simulink model "car_model"  (R2017a)
settings: Solver=ode8  StartTime=0.0  StopTime=tf  FixedStep=1e-3  RelTol=1e-3  AbsTol=1e-6
values from neighbouring files (symbols this model uses):
  sys = kinematic_model(sys)    [load_kin.m]
undefined symbols (not defined in the file or in its folder): L, MAX_DELTA, w, x0
(part 2 of 2)

== matlab function car_model/Vehicle/Steering_model/Efforts/Constrained_efforts ==
  data: in1 input; in2 input; fs output
function fs = ConstrainedEffort(in1,in2)

%    This function was generated by the Symbolic Math Toolbox version 7.2.

%    11-Nov-2020 11:00:39



delta_o = in1(5,:);

f_phi_i = in2(1,:);

f_phi_l = in2(4,:);

f_phi_o = in2(2,:);

f_phi_r = in2(3,:);

p1 = in1(10,:);

p2 = in1(11,:);

p3 = in1(12,:);

p4 = in1(13,:);

phi_i = in1(6,:);

phi_l = in1(9,:);

phi_o = in1(7,:);

phi_r = in1(8,:);

theta = in1(3,:);

t2 = p1.^2;

t3 = tan(theta);

t4 = p4.^2;

t5 = theta.*2.0;

t6 = p3.^2;

t7 = delta_o.*2.0;

t8 = phi_o.*2.0;

t9 = p2.^2;

t10 = t5+t7+t8;

t11 = sin(t10);

t12 = t5+t7-t8;

t13 = sin(t12);

t14 = phi_o.*4.0;

t15 = t5+t7+t14;

t16 = sin(t15);

t17 = sin(t5);

t18 = t5+t7;

t19 = sin(t18);

t20 = phi_l.*2.0;

t21 = phi_l.*4.0;

t22 = -t5+t20;

t23 = sin(t22);

t24 = t5+t20;

t25 = sin(t24);

t26 = phi_l.*3.0;

t27 = phi_r.*2.0;

t28 = phi_r.*4.0;

t29 = delta_o-t14+theta;

t30 = sin(t29);

t31 = delta_o+t14+theta;

t32 = sin(t31);

t33 = phi_o.*3.0;

t34 = t3.*(3.0./2.0);

t35 = t34+9.0./2.0;

t36 = 1.0./t35;

t37 = t3.*t36.*(9.0./2.0);

t38 = atan(t37);

t39 = t38.*2.0;

t40 = delta_o+theta;

t41 = sin(t40);

t42 = phi_i.*4.0;

t43 = t3.*t36.*(2.7e1./4.0);

t44 = t43+9.0./2.0;

t45 = 1.0./t44.^2;

t46 = t21+theta;

t47 = sin(t46);

t48 = t5+t7-t14;

t49 = sin(t48);

t50 = sin(t8);

t51 = sin(t14);

t52 = -t5+t27;

t53 = sin(t52);

t54 = t5+t27;

t55 = sin(t54);

t56 = phi_r.*3.0;

t57 = t21-theta;

t58 = sin(t57);

t59 = -t5+t21;

t60 = sin(t59);

t61 = t5+t21;

t62 = sin(t61);

t63 = cos(theta);

t64 = sin(theta);

t65 = phi_i.*2.0;

t69 = cos(t39);

t70 = t69.*(9.0./2.0);

t71 = sin(t39);

t72 = t71.*(3.0./2.0);

t66 = t70+t72+9.0./2.0;

t67 = t5+t39+t65;

t68 = sin(t67);

t73 = t66.^2;

t74 = cos(t7);

t75 = t74.*(9.0./2.0);

t76 = sin(t7);

t79 = t76.*(3.0./2.0);

t77 = t75-t79+9.0./2.0;

t78 = 1.0./t77.^2;

t80 = t5+t39+t42;

t81 = sin(t80);

t82 = t5+t39;

t83 = sin(t82);

t84 = t38-t42+theta;

t85 = sin(t84);

t86 = t38+t42+theta;

t87 = sin(t86);

t88 = t28+theta;

t89 = sin(t88);

t90 = t38+theta;

t91 = sin(t90);

t92 = 1.0./t44;

t93 = t28-theta;

t94 = sin(t93);

t95 = -t5+t28;

t96 = sin(t95);

t97 = t5+t28;

t98 = sin(t97);

t99 = t5+t39-t65;

t100 = sin(t99);

t101 = 1.0./t77;

t102 = t5+t39-t42;

t103 = sin(t102);

t104 = t3.^2;

t105 = 1.0./t35.^2;

t106 = t104.*t105.*(8.1e1./4.0);

t107 = t106+1.0;

t108 = 1.0./sqrt(t107);

t110 = t108.*9.0;

t111 = t3.*t36.*t108.*(2.7e1./4.0);

t109 = t110-t111;

t112 = cos(delta_o);

t113 = 1.0./t112.^2;

t114 = 1.0./t107;

t115 = t109.^2;

t116 = t110+t111;

t117 = 1.0./t116.^2;

t118 = phi_i.*3.0;

t119 = 1.0./t112;

t120 = 1.0./t116;

t121 = sin(t65);

t122 = sin(t42);

t123 = phi_o+t5+t7;

t124 = sin(t123);

t125 = t6.*t124.*3.888459953911314e-2;

t126 = delta_o+phi_o+theta;

t127 = sin(t126);

t128 = -phi_o+t5+t7;

t129 = sin(t128);

t130 = t6.*t129.*3.888459953911314e-2;

t131 = t2.*t16.*6.480766589852189e-3;

t132 = t9.*t49.*6.480766589852189e-3;

t133 = t9.*t16.*6.480766589852189e-3;

t134 = t5+t7+t33;

t135 = sin(t134);

t136 = t2.*t19.*3.888459953911314e-2;

t137 = t9.*t19.*3.888459953911314e-2;

t138 = t6.*t19.*5.184613271881752e-2;

t139 = delta_o-phi_o+theta;

t140 = sin(t139);

t141 = t2.*t30.*1.296153317970438e-2;

t142 = t2.*t32.*1.296153317970438e-2;

t143 = t9.*t30.*1.296153317970438e-2;

t144 = t9.*t32.*1.296153317970438e-2;

t145 = delta_o-t33+theta;

t146 = sin(t145);

t147 = delta_o+t33+theta;

t148 = sin(t147);

t149 = t2.*t81.*6.480766589852189e-3;

t150 = t2.*t83.*3.888459953911314e-2;

t151 = t2.*t85.*1.296153317970438e-2;

t152 = t2.*t87.*1.296153317970438e-2;

t153 = t9.*t73.*t78.*t103.*6.480766589852189e-3;

t154 = t9.*t73.*t78.*t81.*6.480766589852189e-3;

t155 = t9.*t73.*t78.*t83.*3.888459953911314e-2;

t156 = t9.*t73.*t78.*t85.*1.296153317970438e-2;

t157 = t9.*t73.*t78.*t87.*1.296153317970438e-2;

t158 = p1.*p2.*t66.*t101.*t103.*1.296153317970438e-2;

t159 = p1.*p2.*t66.*t81.*t101.*1.296153317970438e-2;

t160 = p1.*p2.*t66.*t83.*t101.*7.776919907822627e-2;

t161 = p1.*p2.*t66.*t85.*t101.*2.592306635940876e-2;

t162 = p1.*p2.*t66.*t87.*t101.*2.592306635940876e-2;

t163 = t6.*t83.*t113.*t114.*t115.*t117.*5.184613271881752e-2;

t164 = -phi_i+t38+theta;

t165 = sin(t164);

t166 = t38+t118+theta;

t167 = sin(t166);

t168 = phi_i+t5+t39;

t169 = sin(t168);

t170 = t6.*t113.*t114.*t115.*t117.*t169.*3.888459953911314e-2;

t171 = phi_i+t38+theta;

t172 = sin(t171);

t173 = -phi_i+t5+t39;

t174 = sin(t173);

t175 = t6.*t113.*t114.*t115.*t117.*t174.*3.888459953911314e-2;

t176 = t5+t39-t118;

t177 = sin(t176);

t178 = t5+t39+t118;

t179 = sin(t178);

t180 = p1.*p3.*t108.*t109.*t119.*t120.*t121.*1.03692265437635e-1;

t181 = p1.*p3.*t108.*t109.*t119.*t120.*t122.*1.555383981564525e-1;

t182 = p1.*p3.*t100.*t108.*t109.*t119.*t120.*5.184613271881752e-2;

t183 = p1.*p3.*t81.*t108.*t109.*t119.*t120.*2.592306635940876e-2;

t184 = p1.*p3.*t87.*t108.*t109.*t119.*t120.*1.03692265437635e-1;

t185 = p2.*p3.*t66.*t101.*t108.*t109.*t119.*t120.*t121.*1.03692265437635e-1;

t186 = p2.*p3.*t66.*t101.*t108.*t109.*t119.*t120.*t122.*1.555383981564525e-1;

t187 = p2.*p3.*t66.*t100.*t101.*t108.*t109.*t119.*t120.*5.184613271881752e-2;

t188 = p2.*p3.*t66.*t81.*t101.*t108.*t109.*t119.*t120.*2.592306635940876e-2;

t189 = p2.*p3.*t66.*t87.*t101.*t108.*t109.*t119.*t120.*1.03692265437635e-1;

t190 = p1.*p3.*t13.*5.184613271881752e-2;

t191 = p1.*p2.*t49.*1.296153317970438e-2;

t192 = p1.*p2.*t16.*1.296153317970438e-2;

t193 = p2.*p3.*t13.*5.184613271881752e-2;

t194 = p1.*p3.*t16.*2.592306635940876e-2;

t195 = p2.*p3.*t16.*2.592306635940876e-2;

t196 = p1.*p3.*t50.*1.03692265437635e-1;

t197 = p2.*p3.*t50.*1.03692265437635e-1;

t198 = p1.*p3.*t51.*1.555383981564525e-1;

t199 = p2.*p3.*t51.*1.555383981564525e-1;

t200 = p1.*p2.*t19.*7.776919907822627e-2;

t201 = p1.*p2.*t30.*2.592306635940876e-2;

t202 = p1.*p2.*t32.*2.592306635940876e-2;

t203 = p1.*p3.*t32.*1.03692265437635e-1;

t204 = p2.*p3.*t32.*1.03692265437635e-1;

t205 = sin(t33);

t206 = sin(delta_o);

t207 = cos(t5);

t208 = sin(phi_o);

t209 = sin(t118);

t210 = sin(phi_i);

t211 = cos(t65);

t212 = cos(t8);

t213 = t39+theta;

t214 = t63.*(3.0./4.0);

t215 = t64.*(9.0./2.0);

t216 = cos(t213);

t217 = sin(t213);

t218 = t63.*(9.0./2.0);

t219 = t64.*(3.0./4.0);

t220 = sin(phi_r);

t221 = t220.^2;

t222 = cos(phi_r);

t223 = t222.^2;

t224 = t63.^2;

t225 = t64.^2;

t226 = sin(phi_l);

t227 = t226.^2;

t228 = cos(phi_l);

t229 = t228.^2;

fs = [t125+t130+t131+t132+t133+t136+t137+t138+t141+t142+t143+t144+t149+t150+t151+t152+t153+t154+t155+t156+t157+t158+t159+t160+t161+t162+t163+t170+t175+t180+t181+t182+t183+t184+t185+t186+t187+t188+t189+t190+t191+t192+t193+t194+t195+t196+t197+t198+t199+t200+t201+t202+t203+t204-t2.*t11.*2.592306635940876e-2-t6.*t11.*2.592306635940876e-2+t2.*t17.*7.776919907822627e-2-t6.*t13.*2.592306635940876e-2-t9.*t11.*2.592306635940876e-2+t4.*t17.*5.184613271881752e-2-t9.*t13.*2.592306635940876e-2+t2.*t23.*2.592306635940876e-2-t2.*t25.*2.592306635940876e-2+t4.*t23.*2.592306635940876e-2-t4.*t25.*2.592306635940876e-2-t2.*t41.*2.592306635940876e-2+t2.*t47.*1.296153317970438e-2-t9.*t41.*2.592306635940876e-2+t2.*t53.*2.592306635940876e-2-t2.*t55.*2.592306635940876e-2-t2.*t58.*1.296153317970438e-2-t2.*t60.*6.480766589852189e-3+t2.*t62.*6.480766589852189e-3-t2.*t64.*5.184613271881752e-2-t2.*t68.*2.592306635940876e-2+t2.*t89.*1.296153317970438e-2-t2.*t91.*2.592306635940876e-2-t2.*t94.*1.296153317970438e-2-t2.*t96.*6.480766589852189e-3+t2.*t98.*6.480766589852189e-3-t6.*t127.*2.592306635940876e-2-t6.*t135.*3.888459953911314e-2-t6.*t140.*2.592306635940876e-2-t6.*t146.*7.776919907822627e-2-t6.*t148.*7.776919907822627e-2-t2.*sin(phi_o.*-2.0+t5+t7).*2.592306635940876e-2+t2.*sin(phi_o.*-4.0+t5+t7).*6.480766589852189e-3-t6.*sin(phi_o.*-3.0+t5+t7).*3.888459953911314e-2-t2.*sin(phi_i.*-2.0+t5+t39).*2.592306635940876e-2+t2.*sin(phi_i.*-4.0+t5+t39).*6.480766589852189e-3+t4.*sin(phi_l+t5).*3.888459953911314e-2-t4.*sin(phi_l+theta).*2.592306635940876e-2-t4.*sin(t5+t26).*3.888459953911314e-2-t4.*sin(t26+theta).*7.776919907822627e-2-t4.*sin(phi_l-t5).*3.888459953911314e-2+t4.*sin(phi_l-theta).*2.592306635940876e-2+t4.*sin(-t5+t26).*3.888459953911314e-2+t4.*sin(t26-theta).*7.776919907822627e-2-t4.*t45.*sin(t5+t56).*7.87413140667041e-1-t4.*t45.*sin(t56+theta).*1.574826281334082+p1.*p4.*sin(t20).*1.03692265437635e-1+p1.*p4.*sin(t21).*1.555383981564525e-1-t4.*t45.*sin(phi_r-t5).*7.87413140667041e-1+t4.*t45.*sin(phi_r-theta).*5.249420937780273e-1+t4.*t45.*sin(-t5+t56).*7.87413140667041e-1+t4.*t45.*sin(t56-theta).*1.574826281334082-t2.*t64.*(t218+t219).*4.24125e3-p1.*p2.*t11.*5.184613271881752e-2-p1.*p3.*t11.*5.184613271881752e-2-p1.*p2.*t13.*5.184613271881752e-2-p2.*p3.*t11.*5.184613271881752e-2-p1.*p4.*t23.*5.184613271881752e-2-p1.*p4.*t25.*5.184613271881752e-2-p1.*p3.*t30.*1.03692265437635e-1-p2.*p3.*t30.*1.03692265437635e-1-p1.*p2.*t41.*5.184613271881752e-2+p1.*p4.*t47.*1.03692265437635e-1-p1.*p3.*t49.*2.592306635940876e-2-p2.*p3.*t49.*2.592306635940876e-2+p1.*p4.*t58.*1.03692265437635e-1+p1.*p4.*t60.*2.592306635940876e-2+p1.*p4.*t62.*2.592306635940876e-2+t4.*t17.*t45.*1.049884187556055+t4.*t45.*t53.*5.249420937780273e-1-t4.*t45.*t55.*5.249420937780273e-1-t2.*t63.*(t214-t215).*4.24125e3+t4.*t45.*sin(phi_r+t5).*7.87413140667041e-1-t4.*t45.*sin(phi_r+theta).*5.249420937780273e-1-p1.*p4.*t53.*t92.*2.333075972346788e-1-p1.*p4.*t55.*t92.*2.333075972346788e-1+p1.*p4.*t89.*t92.*4.666151944693576e-1+p1.*p4.*t92.*t94.*4.666151944693576e-1+p1.*p4.*t92.*t96.*1.166537986173394e-1+p1.*p4.*t92.*t98.*1.166537986173394e-1-t9.*t68.*t73.*t78.*2.592306635940876e-2-t9.*t73.*t78.*t91.*2.592306635940876e-2-t9.*t73.*t78.*t100.*2.592306635940876e-2+p1.*p4.*t92.*sin(t27).*4.666151944693576e-1+p1.*p4.*t92.*sin(t28).*6.999227917040365e-1-p1.*p2.*t66.*t68.*t101.*5.184613271881752e-2-p1.*p2.*t66.*t91.*t101.*5.184613271881752e-2-p1.*p2.*t66.*t100.*t101.*5.184613271881752e-2-t6.*t68.*t113.*t114.*t115.*t117.*2.592306635940876e-2-t6.*t100.*t113.*t114.*t115.*t117.*2.592306635940876e-2-t6.*t113.*t114.*t115.*t117.*t165.*2.592306635940876e-2-t6.*t113.*t114.*t115.*t117.*t167.*7.776919907822627e-2-t6.*t113.*t114.*t115.*t117.*t172.*2.592306635940876e-2-t6.*t113.*t114.*t115.*t117.*t177.*3.888459953911314e-2-t6.*t113.*t114.*t115.*t117.*t179.*3.888459953911314e-2-t6.*t113.*t114.*t115.*t117.*sin(phi_i.*-3.0+t38+theta).*7.776919907822627e-2-p1.*p3.*t68.*t108.*t109.*t119.*t120.*5.184613271881752e-2-p1.*p3.*t85.*t108.*t109.*t119.*t120.*1.03692265437635e-1-p1.*p3.*t103.*t108.*t109.*t119.*t120.*2.592306635940876e-2-p2.*p3.*t66.*t68.*t101.*t108.*t109.*t119.*t120.*5.184613271881752e-2-p2.*p3.*t66.*t85.*t101.*t108.*t109.*t119.*t120.*1.03692265437635e-1-p2.*p3.*t66.*t101.*t103.*t108.*t109.*t119.*t120.*2.592306635940876e-2;t125+t130+t131+t132+t133+t136+t137+t138+t141+t142+t143+t144+t190+t191+t192+t193+t194+t195+t196+t197+t198+t199+t200+t201+t202+t203+t204-t2.*t11.*2.592306635940876e-2-t2.*t13.*2.592306635940876e-2-t6.*t11.*2.592306635940876e-2-t6.*t13.*2.592306635940876e-2-t9.*t11.*2.592306635940876e-2-t9.*t13.*2.592306635940876e-2-t2.*t41.*2.592306635940876e-2-t9.*t41.*2.592306635940876e-2+t2.*t49.*6.480766589852189e-3-t6.*t127.*2.592306635940876e-2-t6.*t135.*3.888459953911314e-2-t6.*t140.*2.592306635940876e-2-t6.*t146.*7.776919907822627e-2-t6.*t148.*7.776919907822627e-2-t6.*sin(t5+t7-t33).*3.888459953911314e-2+t66.*t101.*(t149+t150+t151+t152+t153+t154+t155+t156+t157+t158+t159+t160+t161+t162+t163+t170+t175+t180+t181+t182+t183+t184+t185+t186+t187+t188+t189-t2.*t68.*2.592306635940876e-2-t2.*t91.*2.592306635940876e-2-t2.*t100.*2.592306635940876e-2+t2.*t103.*6.480766589852189e-3-t9.*t68.*t73.*t78.*2.592306635940876e-2-t9.*t73.*t78.*t91.*2.592306635940876e-2-t9.*t73.*t78.*t100.*2.592306635940876e-2-p1.*p2.*t66.*t68.*t101.*5.184613271881752e-2-p1.*p2.*t66.*t91.*t101.*5.184613271881752e-2-p1.*p2.*t66.*t100.*t101.*5.184613271881752e-2-t6.*t68.*t113.*t114.*t115.*t117.*2.592306635940876e-2-t6.*t100.*t113.*t114.*t115.*t117.*2.592306635940876e-2-t6.*t113.*t114.*t115.*t117.*t165.*2.592306635940876e-2-t6.*t113.*t114.*t115.*t117.*t167.*7.776919907822627e-2-t6.*t113.*t114.*t115.*t117.*t172.*2.592306635940876e-2-t6.*t113.*t114.*t115.*t117.*t177.*3.888459953911314e-2-t6.*t113.*t114.*t115.*t117.*t179.*3.888459953911314e-2-t6.*t113.*t114.*t115.*t117.*sin(t38-t118+theta).*7.776919907822627e-2-p1.*p3.*t68.*t108.*t109.*t119.*t120.*5.184613271881752e-2-p1.*p3.*t85.*t108.*t109.*t119.*t120.*1.03692265437635e-1-p1.*p3.*t103.*t108.*t109.*t119.*t120.*2.592306635940876e-2-p2.*p3.*t66.*t68.*t101.*t108.*t109.*t119.*t120.*5.184613271881752e-2-p2.*p3.*t66.*t85.*t101.*t108.*t109.*t119.*t120.*1.03692265437635e-1-p2.*p3.*t66.*t101.*t103.*t108.*t109.*t119.*t120.*2.592306635940876e-2)-p1.*p2.*t11.*5.184613271881752e-2-p1.*p3.*t11.*5.184613271881752e-2-p1.*p2.*t13.*5.184613271881752e-2-p2.*p3.*t11.*5.184613271881752e-2-p1.*p3.*t30.*1.03692265437635e-1-p2.*p3.*t30.*1.03692265437635e-1-p1.*p2.*t41.*5.184613271881752e-2-p1.*p3.*t49.*2.592306635940876e-2-p2.*p3.*t49.*2.592306635940876e-2;f_phi_o-t2.*t50.*5.184613271881752e-2-t2.*t51.*7.776919907822627e-2-t6.*t50.*5.184613271881752e-2-t9.*t50.*5.184613271881752e-2-t9.*t51.*7.776919907822627e-2-p1.*p2.*t50.*1.03692265437635e-1-p1.*p2.*t51.*1.555383981564525e-1-p1.*p3.*t17.*t74.*1.03692265437635e-1-p2.*p3.*t17.*t74.*1.03692265437635e-1-p1.*p3.*t76.*t207.*1.03692265437635e-1-p2.*p3.*t76.*t207.*1.03692265437635e-1-t2.*t17.*t50.*t76.*5.184613271881752e-2+t2.*t17.*t51.*t76.*2.592306635940876e-2-t6.*t17.*t50.*t76.*5.184613271881752e-2-t9.*t17.*t50.*t76.*5.184613271881752e-2+t9.*t17.*t51.*t76.*2.592306635940876e-2-t2.*t51.*t63.*t112.*1.03692265437635e-1-t9.*t51.*t63.*t112.*1.03692265437635e-1+t2.*t17.*t76.*t205.*5.184613271881752e-2-t2.*t17.*t76.*t208.*1.555383981564525e-1+t9.*t17.*t76.*t205.*5.184613271881752e-2-t9.*t17.*t76.*t208.*1.555383981564525e-1+t2.*t51.*t64.*t206.*1.03692265437635e-1+t9.*t51.*t64.*t206.*1.03692265437635e-1+t2.*t50.*t74.*t207.*5.184613271881752e-2-t2.*t51.*t74.*t207.*2.592306635940876e-2+t6.*t50.*t74.*t207.*5.184613271881752e-2+t9.*t50.*t74.*t207.*5.184613271881752e-2-t9.*t51.*t74.*t207.*2.592306635940876e-2-t2.*t63.*t112.*t205.*5.184613271881752e-2-t2.*t63.*t112.*t208.*5.184613271881752e-2-t9.*t63.*t112.*t205.*5.184613271881752e-2-t9.*t63.*t112.*t208.*5.184613271881752e-2+t2.*t64.*t205.*t206.*5.184613271881752e-2+t2.*t64.*t206.*t208.*5.184613271881752e-2+t9.*t64.*t205.*t206.*5.184613271881752e-2+t9.*t64.*t206.*t208.*5.184613271881752e-2-t2.*t74.*t205.*t207.*5.184613271881752e-2+t2.*t74.*t207.*t208.*1.555383981564525e-1-t9.*t74.*t205.*t207.*5.184613271881752e-2+t9.*t74.*t207.*t208.*1.555383981564525e-1+f_phi_i.*t108.*t109.*t119.*t120-p1.*p2.*t17.*t50.*t76.*1.03692265437635e-1+p1.*p2.*t17.*t51.*t76.*5.184613271881752e-2-p1.*p2.*t51.*t63.*t112.*2.073845308752701e-1+p1.*p2.*t17.*t76.*t205.*1.03692265437635e-1-p1.*p2.*t17.*t76.*t208.*3.110767963129051e-1+p1.*p3.*t17.*t74.*t212.*1.03692265437635e-1+p2.*p3.*t17.*t74.*t212.*1.03692265437635e-1+p1.*p2.*t51.*t64.*t206.*2.073845308752701e-1+p1.*p2.*t50.*t74.*t207.*1.03692265437635e-1-p1.*p2.*t51.*t74.*t207.*5.184613271881752e-2-p1.*p2.*t63.*t112.*t205.*1.03692265437635e-1-p1.*p2.*t63.*t112.*t208.*1.03692265437635e-1+p1.*p2.*t64.*t205.*t206.*1.03692265437635e-1+p1.*p2.*t64.*t206.*t208.*1.03692265437635e-1-p1.*p2.*t74.*t205.*t207.*1.03692265437635e-1+p1.*p2.*t74.*t207.*t208.*3.110767963129051e-1+p1.*p3.*t76.*t207.*t212.*1.03692265437635e-1+p2.*p3.*t76.*t207.*t212.*1.03692265437635e-1-t108.*t109.*t119.*t120.*(t2.*t121.*5.184613271881752e-2+t2.*t122.*7.776919907822627e-2+t2.*t17.*t71.*t121.*5.184613271881752e-2-t2.*t17.*t71.*t122.*2.592306635940876e-2+t9.*t73.*t78.*t121.*5.184613271881752e-2+t9.*t73.*t78.*t122.*7.776919907822627e-2+t2.*t63.*t108.*t122.*1.03692265437635e-1-t2.*t17.*t71.*t209.*5.184613271881752e-2+t2.*t17.*t71.*t210.*1.555383981564525e-1+t2.*t63.*t108.*t209.*5.184613271881752e-2+t2.*t63.*t108.*t210.*5.184613271881752e-2-t2.*t69.*t121.*t207.*5.184613271881752e-2+t2.*t69.*t122.*t207.*2.592306635940876e-2+t2.*t69.*t207.*t209.*5.184613271881752e-2-t2.*t69.*t207.*t210.*1.555383981564525e-1+p1.*p2.*t66.*t101.*t121.*1.03692265437635e-1+p1.*p2.*t66.*t101.*t122.*1.555383981564525e-1-t2.*t3.*t36.*t64.*t108.*t122.*4.666151944693576e-1+t9.*t17.*t71.*t73.*t78.*t121.*5.184613271881752e-2-t9.*t17.*t71.*t73.*t78.*t122.*2.592306635940876e-2-t2.*t3.*t36.*t64.*t108.*t209.*2.333075972346788e-1-t2.*t3.*t36.*t64.*t108.*t210.*2.333075972346788e-1+t9.*t63.*t73.*t78.*t108.*t122.*1.03692265437635e-1-t9.*t17.*t71.*t73.*t78.*t209.*5.184613271881752e-2+t9.*t17.*t71.*t73.*t78.*t210.*1.555383981564525e-1+t9.*t63.*t73.*t78.*t108.*t209.*5.184613271881752e-2+t9.*t63.*t73.*t78.*t108.*t210.*5.184613271881752e-2-t9.*t69.*t73.*t78.*t121.*t207.*5.184613271881752e-2+t9.*t69.*t73.*t78.*t122.*t207.*2.592306635940876e-2+t6.*t113.*t114.*t115.*t117.*t121.*5.184613271881752e-2+t9.*t69.*t73.*t78.*t207.*t209.*5.184613271881752e-2-t9.*t69.*t73.*t78.*t207.*t210.*1.555383981564525e-1+p1.*p2.*t17.*t66.*t71.*t101.*t121.*1.03692265437635e-1-p1.*p2.*t17.*t66.*t71.*t101.*t122.*5.184613271881752e-2+p1.*p2.*t63.*t66.*t101.*t108.*t122.*2.073845308752701e-1-p1.*p2.*t17.*t66.*t71.*t101.*t209.*1.03692265437635e-1+p1.*p2.*t17.*t66.*t71.*t101.*t210.*3.110767963129051e-1+p1.*p2.*t63.*t66.*t101.*t108.*t209.*1.03692265437635e-1+p1.*p2.*t63.*t66.*t101.*t108.*t210.*1.03692265437635e-1-p1.*p2.*t66.*t69.*t101.*t121.*t207.*1.03692265437635e-1+p1.*p2.*t66.*t69.*t101.*t122.*t207.*5.184613271881752e-2+p1.*p2.*t66.*t69.*t101.*t207.*t209.*1.03692265437635e-1-p1.*p2.*t66.*t69.*t101.*t207.*t210.*3.110767963129051e-1+p1.*p3.*t17.*t69.*t108.*t109.*t119.*t120.*1.03692265437635e-1+p1.*p3.*t71.*t108.*t109.*t119.*t120.*t207.*1.03692265437635e-1-t3.*t9.*t36.*t64.*t73.*t78.*t108.*t122.*4.666151944693576e-1-t3.*t9.*t36.*t64.*t73.*t78.*t108.*t209.*2.333075972346788e-1-t3.*t9.*t36.*t64.*t73.*t78.*t108.*t210.*2.333075972346788e-1+t6.*t17.*t71.*t113.*t114.*t115.*t117.*t121.*5.184613271881752e-2-t6.*t69.*t113.*t114.*t115.*t117.*t121.*t207.*5.184613271881752e-2-p1.*p2.*t3.*t36.*t64.*t66.*t101.*t108.*t122.*9.332303889387153e-1-p1.*p2.*t3.*t36.*t64.*t66.*t101.*t108.*t209.*4.666151944693576e-1-p1.*p2.*t3.*t36.*t64.*t66.*t101.*t108.*t210.*4.666151944693576e-1-p1.*p3.*t17.*t69.*t108.*t109.*t119.*t120.*t211.*1.03692265437635e-1-p1.*p3.*t71.*t108.*t109.*t119.*t120.*t207.*t211.*1.03692265437635e-1+p2.*p3.*t17.*t66.*t69.*t101.*t108.*t109.*t119.*t120.*1.03692265437635e-1+p2.*p3.*t66.*t71.*t101.*t108.*t109.*t119.*t120.*t207.*1.03692265437635e-1-p2.*p3.*t17.*t66.*t69.*t101.*t108.*t109.*t119.*t120.*t211.*1.03692265437635e-1-p2.*p3.*t66.*t71.*t101.*t108.*t109.*t119.*t120.*t207.*t211.*1.03692265437635e-1)-t2.*t64.*t108.*t119.*t120.*(t216.*(9.0./2.0)-t217.*(3.0./4.0)+t218+t219).*1.46003419575e3+t2.*t63.*t108.*t119.*t120.*(-t214+t215+t216.*(3.0./4.0)+t217.*(9.0./2.0)).*1.46003419575e3;f_phi_l+f_phi_r.*t92.*(9.0./2.0)-t92.*(t2.*t220.*t224.*2.073845308752701e-1-t2.*t220.*t225.*2.073845308752701e-1+t2.*t63.*t220.*t223.*2.073845308752701e-1+t2.*t220.*t221.*t222.*2.073845308752701e-1-t2.*t220.*t221.*t224.*4.147690617505401e-1+t2.*t220.*t222.*t223.*6.221535926258102e-1+t2.*t220.*t221.*t225.*4.147690617505401e-1-t2.*t220.*t222.*t225.*2.073845308752701e-1-t2.*t220.*t223.*t224.*2.073845308752701e-1+t2.*t220.*t223.*t225.*2.073845308752701e-1-p1.*p4.*t63.*t64.*t92.*1.866460777877431+t4.*t45.*t220.*t222.*t225.*4.199536750224219-t2.*t63.*t220.*t221.*t222.*4.147690617505401e-1+t2.*t63.*t220.*t222.*t223.*4.147690617505401e-1-t2.*t220.*t221.*t222.*t224.*6.221535926258102e-1-t2.*t220.*t222.*t223.*t224.*2.073845308752701e-1+p1.*p4.*t63.*t64.*t92.*t221.*3.732921555754861+p1.*p4.*t63.*t64.*t92.*t223.*1.866460777877431).*(9.0./2.0)-t2.*t224.*t226.*2.073845308752701e-1+t2.*t225.*t226.*2.073845308752701e-1+p1.*p4.*t63.*t64.*4.147690617505401e-1-t2.*t63.*t226.*t229.*2.073845308752701e-1+t2.*t224.*t226.*t227.*4.147690617505401e-1-t2.*t225.*t226.*t227.*4.147690617505401e-1+t2.*t224.*t226.*t229.*2.073845308752701e-1+t2.*t225.*t226.*t228.*2.073845308752701e-1-t2.*t225.*t226.*t229.*2.073845308752701e-1-t2.*t226.*t227.*t228.*2.073845308752701e-1-t4.*t225.*t226.*t228.*2.073845308752701e-1-t2.*t226.*t228.*t229.*6.221535926258102e-1-p1.*p4.*t63.*t64.*t227.*8.295381235010802e-1-p1.*p4.*t63.*t64.*t229.*4.147690617505401e-1+t2.*t63.*t226.*t227.*t228.*4.147690617505401e-1-t2.*t63.*t226.*t228.*t229.*4.147690617505401e-1+t2.*t224.*t226.*t227.*t228.*6.221535926258102e-1+t2.*t224.*t226.*t228.*t229.*2.073845308752701e-1];

end

== matlab function car_model/Vehicle/Steering_model/Mass_block/H ==
  data: C_matrix input; H output; M input
function H = ConstrinedMassMatrix(C_matrix, M)
% MASSMATRIX
%    This function was generated by the Symbolic Math Toolbox version 7.2.
%    16-Oct-2020 11:55:07

    H = C_matrix'*M*C_matrix;
end

== matlab function car_model/Vehicle/Steering_model/Mass_block/invH ==
  data: matrix input; inv_matrix output
function inv_matrix = matrix_inverse(matrix)
% MASSMATRIX
%    This function was generated by the Symbolic Math Toolbox version 7.2.
%    16-Oct-2020 11:55:07

    inv_matrix = inv(matrix);
end

== matlab function car_model/Vehicle/Steering_model/Mass_block/inverse_matrix_ ==
  data: matrix input; inv_matrix output
function inv_matrix = matrix_inverse(matrix)
% MASSMATRIX
%    This function was generated by the Symbolic Math Toolbox version 7.2.
%    16-Oct-2020 11:55:07

    inv_matrix = inv(matrix);
end

== matlab function car_model/Vehicle/Steering_model/Mass_block/square_root_M ==
  data: matrix input; square_root_matrix output
function square_root_matrix = matrix_square_root(matrix)
% MASSMATRIX
%    This function was generated by the Symbolic Math Toolbox version 7.2.
%    16-Oct-2020 11:55:07

    square_root_matrix = real(sqrtm(matrix));
end

== matlab function car_model/Vehicle/Steering_model/Mass_block/inverse_matrix ==
  data: matrix input; inv_matrix output
function inv_matrix = matrix_inverse(matrix)
% MASSMATRIX
%    This function was generated by the Symbolic Math Toolbox version 7.2.
%    16-Oct-2020 11:55:07

    inv_matrix = inv(matrix);
end

== matlab function car_model/Vehicle/Steering_model/Auxiliary_matrices/C_p ==
  data: in1 input; qp output
function qp = KinematicVector(in1)

%    This function was generated by the Symbolic Math Toolbox version 7.2.

%    11-Nov-2020 10:59:48



delta_o = in1(5,:);

p1 = in1(10,:);

p2 = in1(11,:);

p3 = in1(12,:);

p4 = in1(13,:);

theta = in1(3,:);

t2 = tan(theta);

t3 = t2.^2;

t4 = t2.*(3.0./2.0);

t5 = t4+9.0./2.0;

t6 = 1.0./t5.^2;

t7 = t3.*t6.*(8.1e1./4.0);

t8 = t7+1.0;

t9 = 1.0./sqrt(t8);

t10 = 1.0./t5;

t11 = t2.*t10.*(9.0./2.0);

t12 = atan(t11);

t13 = t12.*2.0;

t14 = t13+theta;

t15 = cos(theta);

t16 = t15.*(9.0./2.0);

t17 = sin(theta);

t18 = t17.*(3.0./4.0);

t19 = cos(delta_o);

t20 = 1.0./t19;

t21 = t9.*9.0;

t22 = t2.*t9.*t10.*(2.7e1./4.0);

t23 = t21+t22;

t24 = 1.0./t23;

t25 = cos(t14);

t26 = sin(t14);

t27 = t15.*(3.0./4.0);

t28 = t17.*(9.0./2.0);

t29 = delta_o.*2.0;

qp = [p1.*(t16+t18)+p3.*t9.*t20.*t24.*(t16+t18+t25.*(9.0./2.0)-t26.*(3.0./4.0)).*3.442462000000001e-1;-p1.*(t27-t28)+p3.*t9.*t20.*t24.*(t25.*(3.0./4.0)+t26.*(9.0./2.0)-t27+t28).*3.442462000000001e-1;p1;(p2.*(cos(t13).*(9.0./2.0)+sin(t13).*(3.0./2.0)+9.0./2.0))./(cos(t29).*(9.0./2.0)-sin(t29).*(3.0./2.0)+9.0./2.0);p2;p3.*t9.*t20.*t24.*(t21-t22);p3;(p4.*(9.0./2.0))./(t2.*t10.*(2.7e1./4.0)+9.0./2.0);p4];

end
